simulink model "BiCopterModel"  (R2025b)
settings: Solver=VariableStepAuto  StartTime=0.0  StopTime=10.0  RelTol=1e-3
settings Model: Creator=bohdanusatov  LastModifiedBy=bohdanusatov

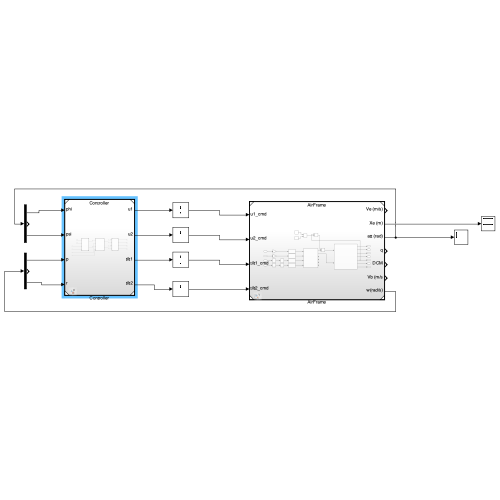
[thumbnail: Simulink's stored preview of the top-level diagram]
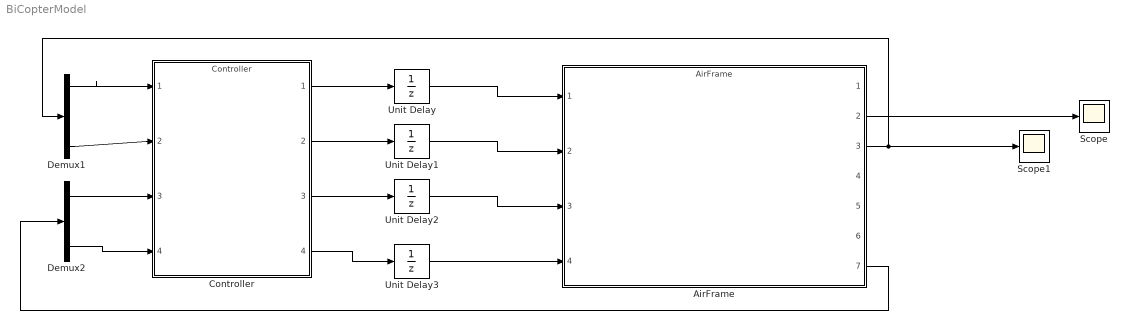
== system BiCopterModel ==
  AirFrame : ModelReference  ModelNameDialog=AirFrame.slx  ModelReferenceVersion=1.8
  Controller : ModelReference  ModelNameDialog=Controller.slx  ModelReferenceVersion=1.12
  Demux1 : Demux  Outputs=3
  Demux2 : Demux  Outputs=3
  Scope : Scope
      settings: ActiveDisplayYMinimum=-485.20330839668145  ActiveDisplayYMaximum=58.770855108923293
  Scope1 : Scope
      settings: ActiveDisplayYMinimum=-0.12742592162415536  ActiveDisplayYMaximum=0.12526954684712835
  Unit Delay{,1..3} (4 alike) : UnitDelay  SampleTime=-1  HasFrameUpgradeWarning=on
  wires:
  Controller/1 -> Unit Delay/1
  Demux1/1 -> Controller/1
  Demux1/3 -> Controller/2
  AirFrame/7 -> Demux2/1
  Demux2/1 -> Controller/3
  Demux2/3 -> Controller/4
  AirFrame/2 -> Scope/1
  AirFrame/3 -> Demux1/1, Scope1/1
  Unit Delay/1 -> AirFrame/1
  Controller/2 -> Unit Delay1/1
  Controller/3 -> Unit Delay2/1
  Controller/4 -> Unit Delay3/1
  Unit Delay1/1 -> AirFrame/2
  Unit Delay2/1 -> AirFrame/3
  Unit Delay3/1 -> AirFrame/4
